simulink model "modelo_planta_sin_reference"  (R2023b)
settings: Solver=VariableStepAuto  StartTime=0.0  StopTime=50  RelTol=1e-3
undefined symbols (not defined in the file): ah_max, at_max, bcx, bcy, bhb, bhd, bhEb, bhm, bhwu, bt, btb, btd, btm, btw, DiscIntNeverNeededParam, g, h_vec, Hc, ih, it, J_hd_hEb, J_hm_hb, Jtd, Jtm_tb, Kcy, khwu, Ki_v, Kp_v, Kp_x, Ktw, Lh0, lh_0, M_base, magnitude, Mc_max, Ms, Mt, N_h, omega_h, P_nom, rhd, rtd, tau_hm, tau_tm, Thb_Max, ThEb_Max, Thm_0, Thm_Max, titahm_0, titatm_0, Ts2, Ttb_Max, Ttm_0, Ttm_Max, vh_max_unloaded, vlx_0, vly_0, vt_0, vt_max, Wc ... (+15)
libraries: simulink x12, simulink_extras x1
settings Model: Creator=Nahuel  LastModifiedBy=Nahuel

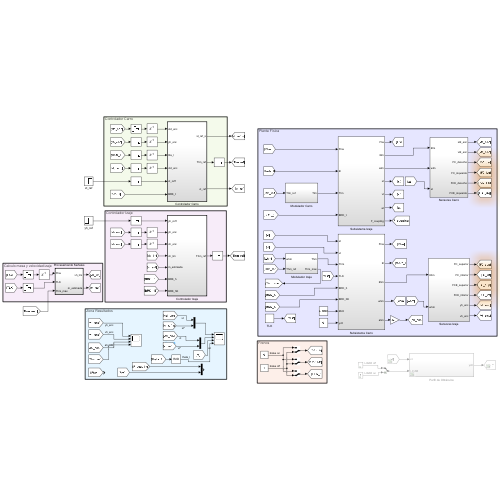
[thumbnail: Simulink's stored preview of the top-level diagram]
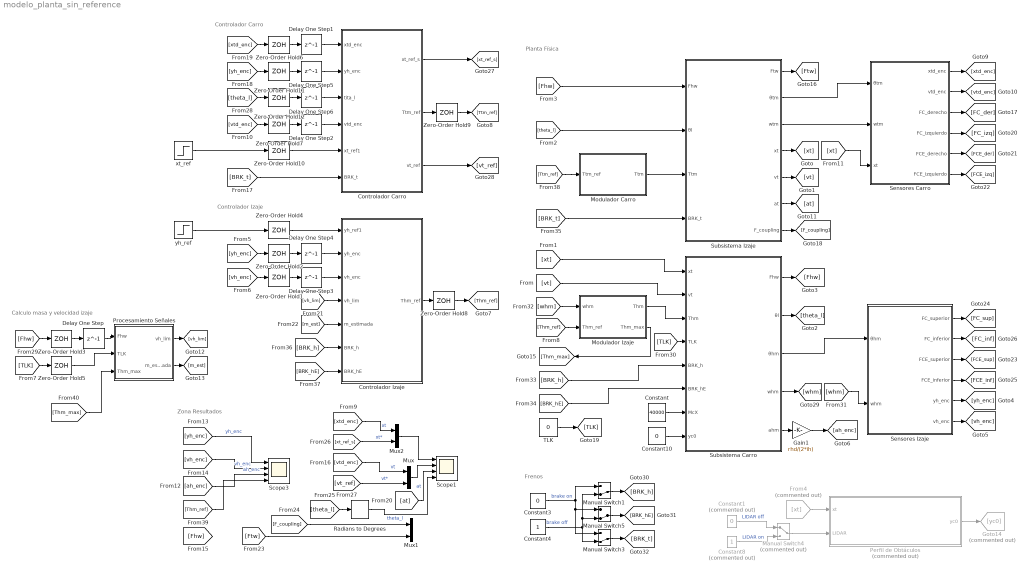
== system modelo_planta_sin_reference ==
  note: Frenos
  note: Controlador Izaje
  note: Calculo masa y velocidad izaje
  note: Controlador Carro
  note: Planta Física
  note: Zona Resultados
  Constant : Constant  Value=40000
  Constant1 : Constant  Commented=on  Value=0
  Constant10 : Constant  Value=0
  Constant3 : Constant  Value=0
  Constant4 : Constant
  Constant8 : Constant  Commented=on
  Controlador Carro : Subsystem  TreatAsAtomicUnit=on  SystemSampleTime=Ts2
  Controlador Izaje : Subsystem  TreatAsAtomicUnit=on  SystemSampleTime=Ts2
  Delay One Step : Delay  DelayLength=1
  Delay One Step1 : Delay  DelayLength=1  InitialCondition=xt_0
  Delay One Step2 : Delay  DelayLength=1  InitialCondition=vt_0
  Delay One Step3 : Delay  DelayLength=1  InitialCondition=whm_0
  Delay One Step4 : Delay  DelayLength=1  InitialCondition=yh_0
  Delay One Step5 : Delay  DelayLength=1  InitialCondition=yh_0
  Delay One Step6 : Delay  DelayLength=1  InitialCondition=0
  From4 : From  Commented=on  GotoTag=xt
  Gain1 : Gain  Gain=rhd/(2*ih)
  Goto14 : Goto  Commented=on  GotoTag=yc0
  Manual Switch1 : ManualSwitch  CurrentSetting=0
  Manual Switch3 : ManualSwitch  CurrentSetting=0
  Manual Switch4 : ManualSwitch  Commented=on
  Manual Switch5 : ManualSwitch  CurrentSetting=0
  Modulador Carro : Subsystem
  Modulador Izaje : Subsystem
  Mux : Mux  Inputs=2
  Mux1 : Mux  Inputs=2
  Mux2 : Mux  Inputs=2
  Perfil de Obtáculos : Subsystem  Commented=on
  Procesamiento Señales : Subsystem  TreatAsAtomicUnit=on  SystemSampleTime=Ts2
  Radians to Degrees : simulink_extras/Transformations/Radians to Degrees
  Scope1 : Scope  NumInputPorts=4
  Scope3 : Scope  NumInputPorts=4
  Sensores Carro : Subsystem
  Sensores Izaje : Subsystem
  Subsistema Carro : Subsystem
  Subsistema Izaje : Subsystem
  TLK : Constant  Value=0
  Zero-Order Hold{1..12} (12 alike) : ZeroOrderHold  SampleTime=Ts2
  xt_ref : Step  Time=0  Before=xt_0  After=0  SampleTime=0
  yh_ref : Step  Time=2  Before=yh_0  After=36.4  SampleTime=0
  wires:
  [Thm_ref] -> Modulador Izaje/2(Thm_ref)
  yh_ref/1 -> Zero-Order Hold4/1
  Constant1/1 -> Manual Switch4/1  "LIDAR off"
  [vt_ref] -> Mux/2  "vt*"
  Zero-Order Hold12/1 -> Delay One Step6/1
  [vh_enc] -> Scope3/2  "vh_enc"
  Sensores Izaje/2(FC_inferior) -> [FC_inf]
  [xt_ref_s] -> Mux2/2  "xt*"
  Controlador Carro/3(vt_ref) -> [vt_ref]
  xt_ref/1 -> Zero-Order Hold10/1
  Zero-Order Hold4/1 -> Controlador Izaje/1(yh_ref1)
  Delay One Step4/1 -> Controlador Izaje/2(yh_enc)
  Sensores Izaje/5(yh_enc) -> [yh_enc]
  [BRK_hE] -> Subsistema Carro/6(BRK_hE)
  Subsistema Carro/1(Fhw) -> [Fhw]
  [xtd_enc] -> Mux2/1  "xt"
  [vh_enc] -> Zero-Order Hold1/1
  Controlador Izaje/1(Thm_ref) -> Zero-Order Hold8/1
  Gain1/1 -> [ah_enc]
  Sensores Carro/1(xtd_enc) -> [xtd_enc]
  [yh_enc] -> Zero-Order Hold11/1
  Delay One Step6/1 -> Controlador Carro/3(tita_l)
  Zero-Order Hold11/1 -> Delay One Step5/1
  [xt] -> Sensores Carro/3(xt)
  [BRK_h] -> Subsistema Carro/5(BRK_h)
  [Ftw] -> Mux1/2
  Sensores Carro/4(FC_izquierdo) -> [FC_izq]
  [theta_l] -> Zero-Order Hold12/1
  Subsistema Carro/4(whm) -> [whm]
  Zero-Order Hold3/1 -> Delay One Step/1
  [m_est] -> Controlador Izaje/5(m_estimada)
  Controlador Carro/1(xt_ref_s) -> [xt_ref_s]
  Zero-Order Hold1/1 -> Delay One Step3/1
  Zero-Order Hold2/1 -> Delay One Step4/1
  Zero-Order Hold6/1 -> Delay One Step1/1
  Mux/1 -> Scope1/2
  Delay One Step/1 -> Procesamiento Señales/1(Fhw)
  Mux2/1 -> Scope1/1
  Subsistema Izaje/3(wtm) -> Sensores Carro/2(wtm)
  [Fhw] -> Zero-Order Hold3/1
  [at] -> Scope1/3  "at"
  Subsistema Izaje/6(at) -> [at]
  [vtd_enc] -> Mux/1  "vt"
  [theta_l] -> Subsistema Izaje/2(θl)
  [vt] -> Subsistema Carro/2(vt)
  [xt] -> Subsistema Carro/1(xt)
  Delay One Step1/1 -> Controlador Carro/1(xtd_enc)
  Procesamiento Señales/2(m_estimada) -> [m_est]
  [ah_enc] -> Scope3/3  "ah_enc"
  [vtd_enc] -> Zero-Order Hold7/1
  Subsistema Carro/5(ahm) -> Gain1/1
  Sensores Carro/2(vtd_enc) -> [vtd_enc]
  [TLK] -> Zero-Order Hold5/1
  Zero-Order Hold8/1 -> [Thm_ref]
  TLK/1 -> [TLK]
  Delay One Step3/1 -> Controlador Izaje/3(vh_enc)
  [vh_lim] -> Controlador Izaje/4(vh_lim)
  Subsistema Izaje/7(F_coupling) -> [F_coupling]
  Procesamiento Señales/1(vh_lim) -> [vh_lim]
  Zero-Order Hold5/1 -> Procesamiento Señales/2(TLK)
  Delay One Step2/1 -> Controlador Carro/4(vtd_enc)
  Zero-Order Hold10/1 -> Controlador Carro/5(xt_ref1)
  [theta_l] -> Radians to Degrees/1
  From4/1 -> Perfil de Obtáculos/1(xt)
  Subsistema Izaje/4(xt) -> [xt]
  [Fhw] -> Subsistema Izaje/1(Fhw)
  [F_coupling] -> Mux1/1
  Sensores Carro/6(FCE_izquierdo) -> [FCE_izq]
  [yh_enc] -> Zero-Order Hold2/1
  Perfil de Obtáculos/1(yc0) -> Goto14/1
  Sensores Izaje/6(vh_enc) -> [vh_enc]
  Constant8/1 -> Manual Switch4/2  "LIDAR on"
  [xtd_enc] -> Zero-Order Hold6/1
  Zero-Order Hold9/1 -> [Ttm_ref]
  Radians to Degrees/1 -> Scope1/4  "theta_l"
  Controlador Carro/2(Ttm_ref) -> Zero-Order Hold9/1
  [TLK] -> Subsistema Carro/4(TLK)
  Subsistema Carro/3(θhm) -> Sensores Izaje/1(θhm)
  Subsistema Izaje/2(θtm) -> Sensores Carro/1(θtm)
  Constant10/1 -> Subsistema Carro/8(yc0)
  Sensores Izaje/4(FCE_inferior) -> [FCE_inf]
  Sensores Izaje/3(FCE_superior) -> [FCE_sup]
  Sensores Izaje/1(FC_superior) -> [FC_sup]
  Manual Switch4/1 -> Perfil de Obtáculos/2(LIDAR)
  Sensores Carro/5(FCE_derecho) -> [FCE_der]
  Zero-Order Hold7/1 -> Delay One Step2/1
  Subsistema Carro/2(θl) -> [theta_l]
  Delay One Step5/1 -> Controlador Carro/2(yh_enc)
  Constant/1 -> Subsistema Carro/7(McX)
  Subsistema Izaje/5(vt) -> [vt]
  Sensores Carro/3(FC_derecho) -> [FC_der]
  Subsistema Izaje/1(Ftw) -> [Ftw]
  [whm] -> Sensores Izaje/2(whm)
  Constant3/1 -> Manual Switch3/1, Manual Switch5/1, Manual Switch1/1  "brake on"
  Constant4/1 -> Manual Switch1/2, Manual Switch5/2, Manual Switch3/2  "brake off"
  Manual Switch1/1 -> [BRK_h]
  Manual Switch5/1 -> [BRK_hE]
  Manual Switch3/1 -> [BRK_t]
  [BRK_t] -> Subsistema Izaje/4(BRK_t)
  [BRK_h] -> Controlador Izaje/6(BRK_h)
  [BRK_hE] -> Controlador Izaje/7(BRK_hE)
  [Ttm_ref] -> Modulador Carro/1(Ttm_ref)
  [BRK_t] -> Controlador Carro/6(BRK_t)
  [yh_enc] -> Scope3/1  "yh_enc"
  [whm] -> Modulador Izaje/1(whm)
  [Thm_ref] -> Scope3/4
  Modulador Carro/1(Ttm) -> Subsistema Izaje/3(Ttm)
  Modulador Izaje/2(Thm_max) -> [Thm_max]
  Modulador Izaje/1(Thm) -> Subsistema Carro/3(Thm)
  [Thm_max] -> Procesamiento Señales/3(Thm_max)

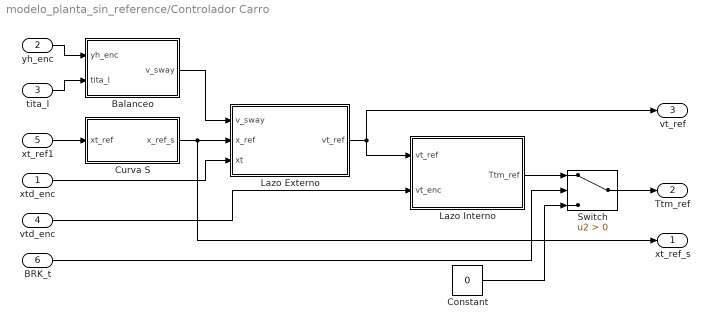
== system modelo_planta_sin_reference/Controlador Carro ==
  xtd_enc : Inport
  yh_enc : Inport  Port=2
  tita_l : Inport  Port=3
  vtd_enc : Inport  Port=4
  xt_ref1 : Inport  Port=5
  BRK_t : Inport  Port=6
  Balanceo : Subsystem
  Constant : Constant  Value=0
  Curva S : Subsystem
  Lazo Externo : Subsystem
  Lazo Interno : Subsystem
  Switch : Switch  Criteria=u2 > Threshold  SaturateOnIntegerOverflow=off  InputSameDT=off
  xt_ref_s : Outport
  Ttm_ref : Outport  Port=2
  vt_ref : Outport  Port=3
  wires:
  Lazo Externo/1(vt_ref) -> vt_ref/1, Lazo Interno/1(vt_ref)
  vtd_enc/1 -> Lazo Interno/2(vt_enc)
  xt_ref1/1 -> Curva S/1(xt_ref)
  Curva S/1(x_ref_s) -> xt_ref_s/1, Lazo Externo/2(x_ref)
  tita_l/1 -> Balanceo/2(tita_l)
  xtd_enc/1 -> Lazo Externo/3(xt)
  Balanceo/1(v_sway) -> Lazo Externo/1(v_sway)
  yh_enc/1 -> Balanceo/1(yh_enc)
  Switch/1 -> Ttm_ref/1
  BRK_t/1 -> Switch/2
  Lazo Interno/1(Ttm_ref) -> Switch/1
  Constant/1 -> Switch/3

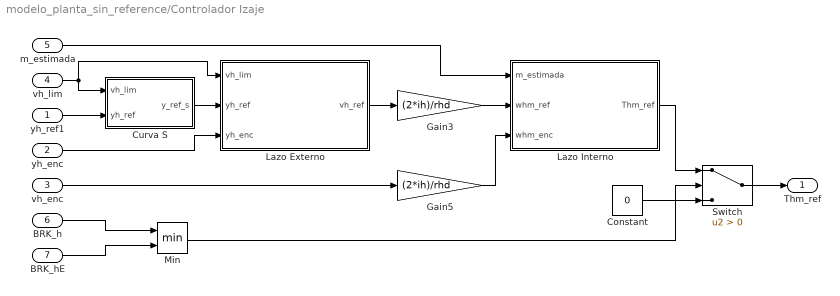
== system modelo_planta_sin_reference/Controlador Izaje ==
  yh_ref1 : Inport
  yh_enc : Inport  Port=2
  vh_enc : Inport  Port=3
  vh_lim : Inport  Port=4
  m_estimada : Inport  Port=5
  BRK_h : Inport  Port=6
  BRK_hE : Inport  Port=7
  Constant : Constant  Value=0
  Curva S : Subsystem
  Gain3 : Gain  Gain=(2*ih)/rhd
  Gain5 : Gain  Gain=(2*ih)/rhd
  Lazo Externo : Subsystem  TreatAsAtomicUnit=on  SystemSampleTime=Ts2
  Lazo Interno : Subsystem  TreatAsAtomicUnit=on  SystemSampleTime=Ts2
  Min : MinMax  Inputs=2
  Switch : Switch  Criteria=u2 > Threshold  SaturateOnIntegerOverflow=off  InputSameDT=off
  Thm_ref : Outport
  wires:
  Lazo Externo/1(vh_ref) -> Gain3/1
  m_estimada/1 -> Lazo Interno/1(m_estimada)
  vh_enc/1 -> Gain5/1
  yh_enc/1 -> Lazo Externo/3(yh_enc)
  Gain5/1 -> Lazo Interno/3(whm_enc)
  yh_ref1/1 -> Curva S/2(yh_ref)
  Gain3/1 -> Lazo Interno/2(whm_ref)
  Curva S/1(y_ref_s) -> Lazo Externo/2(yh_ref)
  BRK_h/1 -> Min/1
  BRK_hE/1 -> Min/2
  Min/1 -> Switch/2
  Switch/1 -> Thm_ref/1
  Lazo Interno/1(Thm_ref) -> Switch/1
  Constant/1 -> Switch/3
  vh_lim/1 -> Curva S/1(vh_lim), Lazo Externo/1(vh_lim)

== system modelo_planta_sin_reference/Modulador Carro ==
  Ttm_ref : Inport
  Constant : Constant  Value=Ttm_Max
  Gain1 : Gain  Gain=-1
  Gain2 : Gain  Gain=1/tau_tm
  Integrator : Integrator  InitialCondition=Ttm_0
  Saturation Dynamic : simulink/Discontinuities/Saturation Dynamic  OutMin=[]  OutMax=[]  OutDataTypeStr=Inherit: Same as second input  OutDataType=fixdt(1, 16)  OutScaling=2^-10  DoSatur=off
  Sum : Sum  Inputs=|+-
  Ttm : Outport
  wires:
  Constant/1 -> Saturation Dynamic/1, Gain1/1
  Gain1/1 -> Saturation Dynamic/3
  Saturation Dynamic/1 -> Sum/1  "Ttm_lim"
  Sum/1 -> Gain2/1
  Gain2/1 -> Integrator/1
  Integrator/1 -> Ttm/1, Sum/2
  Ttm_ref/1 -> Saturation Dynamic/2

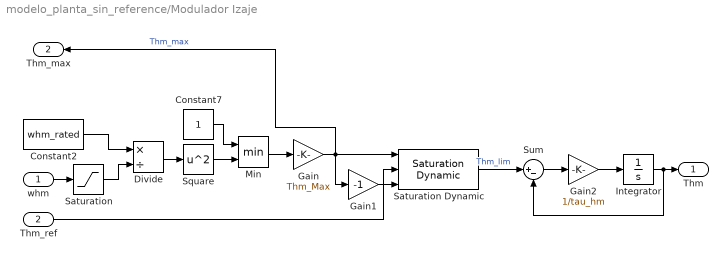
== system modelo_planta_sin_reference/Modulador Izaje ==
  whm : Inport
  Thm_ref : Inport  Port=2
  Constant2 : Constant  Value=whm_rated
  Constant7 : Constant
  Divide : Product  Inputs=*/
  Gain : Gain  Gain=Thm_Max
  Gain1 : Gain  Gain=-1
  Gain2 : Gain  Gain=1/tau_hm
  Integrator : Integrator  InitialCondition=Thm_0
  Min : MinMax  Inputs=2
  Saturation : Saturate  UpperLimit=inf  LowerLimit=whm_rated
  Saturation Dynamic : simulink/Discontinuities/Saturation Dynamic  OutMin=[]  OutMax=[]  OutDataTypeStr=Inherit: Same as second input  OutDataType=fixdt(1, 16)  OutScaling=2^-10  DoSatur=off
  Square : Math  Operator=square
  Sum : Sum  Inputs=|+-
  Thm : Outport
  Thm_max : Outport  Port=2
  wires:
  Constant2/1 -> Divide/1
  Min/1 -> Gain/1
  Constant7/1 -> Min/1
  Gain/1 -> Thm_max/1, Gain1/1, Saturation Dynamic/1  "Thm_max"
  Saturation/1 -> Divide/2
  Square/1 -> Min/2
  Divide/1 -> Square/1
  whm/1 -> Saturation/1
  Gain1/1 -> Saturation Dynamic/3
  Saturation Dynamic/1 -> Sum/1  "Thm_lim"
  Sum/1 -> Gain2/1
  Gain2/1 -> Integrator/1
  Integrator/1 -> Sum/2, Thm/1
  Thm_ref/1 -> Saturation Dynamic/2

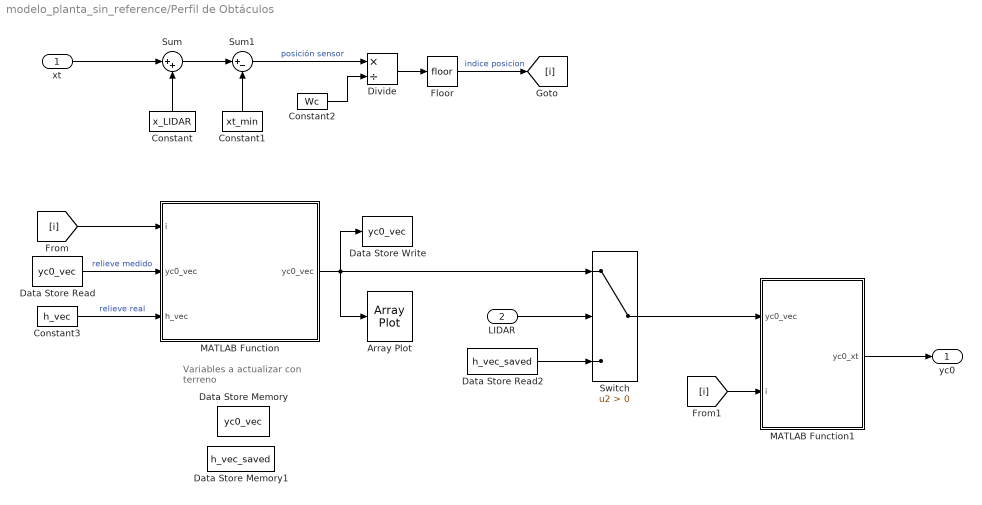
== system modelo_planta_sin_reference/Perfil de Obtáculos ==
  note: Variables a actualizar
      | con terreno
  xt : Inport
  LIDAR : Inport  Port=2
  Array Plot : ArrayPlot  WindowPosition=[1051.000000,310.000000,800.000000,459.000000,]  ScopeFrameLocation=window  YLimits=[-2.5 22.5]
  Constant : Constant  Value=x_LIDAR
  Constant1 : Constant  Value=xt_min
  Constant2 : Constant  Value=Wc
  Constant3 : Constant  Value=h_vec
  Data Store Memory : DataStoreMemory  DataStoreName=yc0_vec  WriteAfterWriteMsg=warning  InitialValue=yc0_vec  ShowAdditionalParam=off
  Data Store Memory1 : DataStoreMemory  DataStoreName=h_vec_saved  WriteAfterWriteMsg=warning  InitialValue=h_vec_saved  ShowAdditionalParam=off
  Data Store Read : DataStoreRead  DataStoreName=yc0_vec  IndexOptions=Index vector (dialog)  Indices=1  OutputSizes=1
  Data Store Read2 : DataStoreRead  DataStoreName=h_vec_saved  IndexOptions=Index vector (dialog)  Indices=1  OutputSizes=1
  Data Store Write : DataStoreWrite  DataStoreName=yc0_vec  IndexOptions=Index vector (dialog)  Indices=1  OutputSizes=1
  Divide : Product  Inputs=*/
  Floor : Rounding
  MATLAB Function : MATLAB Function  TreatAsAtomicUnit=on
  MATLAB Function1 : MATLAB Function  TreatAsAtomicUnit=on
  Sum : Sum  Inputs=|++
  Sum1 : Sum  Inputs=|+-
  Switch : Switch  Criteria=u2 > Threshold  SaturateOnIntegerOverflow=off  InputSameDT=off
  yc0 : Outport
  wires:
  xt/1 -> Sum/1
  Constant/1 -> Sum/2
  Sum/1 -> Sum1/1
  Constant1/1 -> Sum1/2
  Sum1/1 -> Divide/1  "posición sensor"
  Constant2/1 -> Divide/2
  Divide/1 -> Floor/1
  Data Store Read/1 -> MATLAB Function/2("yc0_vec ")  "relieve medido"
  MATLAB Function/1(yc0_vec) -> Array Plot/1, Data Store Write/1, Switch/1
  Constant3/1 -> MATLAB Function/3(h_vec)  "relieve real"
  LIDAR/1 -> Switch/2
  Data Store Read2/1 -> Switch/3
  Switch/1 -> MATLAB Function1/1(yc0_vec)
  MATLAB Function1/1(yc0_xt) -> yc0/1
  Floor/1 -> [i]  "indice posicion"
  [i] -> MATLAB Function/1(i)
  [i] -> MATLAB Function1/2(i)

== system modelo_planta_sin_reference/Procesamiento Señales ==
  Fhw : Inport
  TLK : Inport  Port=2
  Thm_max : Inport  Port=3
  Curva Potencia Original (no anda?) : MATLAB Function  TreatAsAtomicUnit=on
  Curva de Potencia : MATLAB Function  TreatAsAtomicUnit=on
  Estimación de Masa : Subsystem
  vh_lim : Outport
  m_estimada : Outport  Port=2
  wires:
  Estimación de Masa/1(m_estimada) -> Curva de Potencia/1(m_estimada), m_estimada/1
  TLK/1 -> Estimación de Masa/2(TLK)
  Fhw/1 -> Estimación de Masa/1(Fhw)
  Thm_max/1 -> Curva de Potencia/2(Thm_Max)
  Curva de Potencia/1(vh_lim) -> vh_lim/1

== system modelo_planta_sin_reference/Sensores Carro ==
  θtm : Inport
  wtm : Inport  Port=2
  xt : Inport  Port=3
  Encoder Carro : Subsystem
  Fines de carrera carro (rieles) : Subsystem
  xtd_enc : Outport
  vtd_enc : Outport  Port=2
  FC_derecho : Outport  Port=3
  FC_izquierdo : Outport  Port=4
  FCE_derecho : Outport  Port=5
  FCE_izquierdo : Outport  Port=6
  wires:
  Encoder Carro/1(xtd_enc) -> xtd_enc/1
  Fines de carrera carro (rieles)/1(FC_derecho) -> FC_derecho/1
  θtm/1 -> Encoder Carro/1(θtm)
  Fines de carrera carro (rieles)/2(FC_izquierdo) -> FC_izquierdo/1
  Encoder Carro/2(vtd_enc) -> vtd_enc/1
  Fines de carrera carro (rieles)/3(FCE_derecho) -> FCE_derecho/1
  Fines de carrera carro (rieles)/4(FCE_izquierdo) -> FCE_izquierdo/1
  xt/1 -> Fines de carrera carro (rieles)/1(xt)
  wtm/1 -> Encoder Carro/2(wtm)

== system modelo_planta_sin_reference/Sensores Izaje ==
  θhm : Inport
  whm : Inport  Port=2
  Encoder Izaje : Subsystem
  Fines de carrera izaje (tambor) : Subsystem
  FC_superior : Outport
  FC_inferior : Outport  Port=2
  FCE_superior : Outport  Port=3
  FCE_inferior : Outport  Port=4
  yh_enc : Outport  Port=5
  vh_enc : Outport  Port=6
  wires:
  Fines de carrera izaje (tambor)/1(FC_superior) -> FC_superior/1
  whm/1 -> Encoder Izaje/2(whm)
  Fines de carrera izaje (tambor)/4(FCE_inferior) -> FCE_inferior/1
  Fines de carrera izaje (tambor)/2(FC_inferior) -> FC_inferior/1
  Encoder Izaje/2(yh_enc) -> Fines de carrera izaje (tambor)/1(y_enc), yh_enc/1
  θhm/1 -> Encoder Izaje/1(θhm)
  Fines de carrera izaje (tambor)/3(FCE_superior) -> FCE_superior/1
  Encoder Izaje/1(vh_enc) -> vh_enc/1

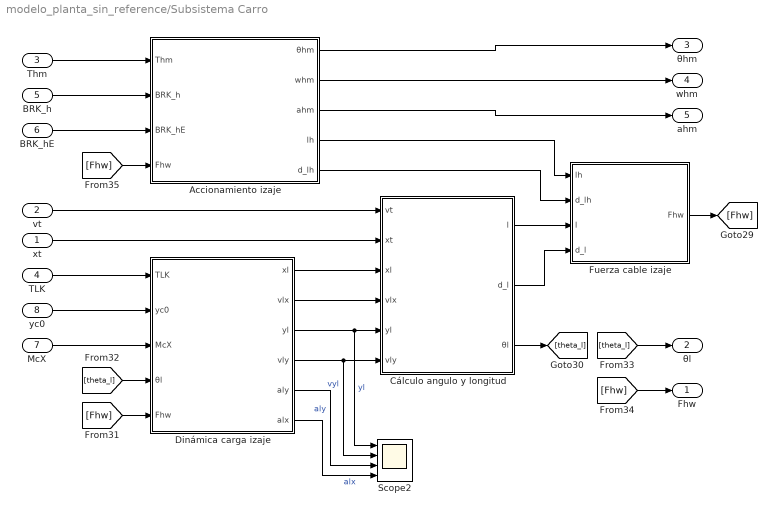
== system modelo_planta_sin_reference/Subsistema Carro ==
  xt : Inport
  vt : Inport  Port=2
  Thm : Inport  Port=3
  TLK : Inport  Port=4
  BRK_h : Inport  Port=5
  BRK_hE : Inport  Port=6
  McX : Inport  Port=7
  yc0 : Inport  Port=8
  Accionamiento izaje : Subsystem
  Cálculo angulo y longitud : Subsystem
  Dinámica carga izaje : Subsystem
  Fuerza cable izaje : Subsystem
  Scope2 : Scope  NumInputPorts=4
  Fhw : Outport
  θl : Outport  Port=2
  θhm : Outport  Port=3
  whm : Outport  Port=4
  ahm : Outport  Port=5
  wires:
  [Fhw] -> Fhw/1
  vt/1 -> Cálculo angulo y longitud/1(vt)
  Accionamiento izaje/4(lh) -> Fuerza cable izaje/1(lh)
  Dinámica carga izaje/5(aly) -> Scope2/3  "aly"
  yc0/1 -> Dinámica carga izaje/2(yc0)
  McX/1 -> Dinámica carga izaje/3(McX)
  Dinámica carga izaje/4(vly) -> Cálculo angulo y longitud/6(vly), Scope2/2  "vyl"
  [Fhw] -> Accionamiento izaje/4(Fhw)
  [theta_l] -> Dinámica carga izaje/4(θl)
  Cálculo angulo y longitud/3(θl) -> [theta_l]
  xt/1 -> Cálculo angulo y longitud/2(xt)
  BRK_h/1 -> Accionamiento izaje/2(BRK_h)
  Dinámica carga izaje/1(xl) -> Cálculo angulo y longitud/3(xl)
  Dinámica carga izaje/2(vlx) -> Cálculo angulo y longitud/4(vlx)
  Accionamiento izaje/3(ahm) -> ahm/1
  Dinámica carga izaje/6(alx) -> Scope2/4  "alx"
  Fuerza cable izaje/1(Fhw) -> [Fhw]
  Cálculo angulo y longitud/1(l) -> Fuerza cable izaje/3(l)
  Accionamiento izaje/1(θhm) -> θhm/1
  [theta_l] -> θl/1
  TLK/1 -> Dinámica carga izaje/1(TLK)
  [Fhw] -> Dinámica carga izaje/5(Fhw)
  Accionamiento izaje/2(whm) -> whm/1
  BRK_hE/1 -> Accionamiento izaje/3(BRK_hE)
  Thm/1 -> Accionamiento izaje/1(Thm)
  Dinámica carga izaje/3(yl) -> Cálculo angulo y longitud/5(yl), Scope2/1  "yl"
  Cálculo angulo y longitud/2(d_l) -> Fuerza cable izaje/4(d_l)
  Accionamiento izaje/5(d_lh) -> Fuerza cable izaje/2(d_lh)

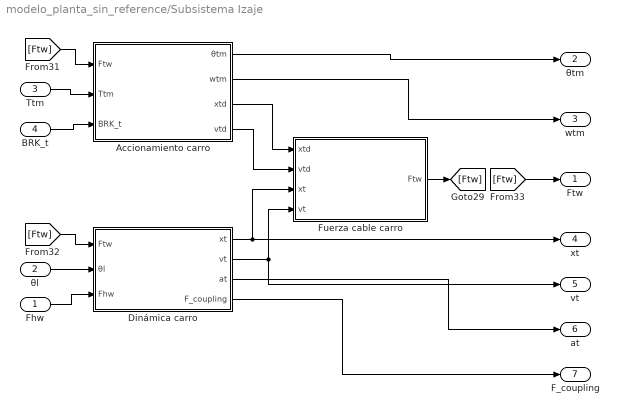
== system modelo_planta_sin_reference/Subsistema Izaje ==
  Fhw : Inport
  θl : Inport  Port=2
  Ttm : Inport  Port=3
  BRK_t : Inport  Port=4
  Accionamiento carro : Subsystem
  Dinámica carro : Subsystem
  Fuerza cable carro : Subsystem
  Ftw : Outport
  θtm : Outport  Port=2
  wtm : Outport  Port=3
  xt : Outport  Port=4
  vt : Outport  Port=5
  at : Outport  Port=6
  F_coupling : Outport  Port=7
  wires:
  [Ftw] -> Accionamiento carro/1(Ftw)
  Accionamiento carro/1(θtm) -> θtm/1
  Dinámica carro/1(xt) -> xt/1, Fuerza cable carro/3(xt)
  BRK_t/1 -> Accionamiento carro/3(BRK_t)
  [Ftw] -> Dinámica carro/1(Ftw)
  θl/1 -> Dinámica carro/2(θl)
  Ttm/1 -> Accionamiento carro/2(Ttm)
  Fuerza cable carro/1(Ftw) -> [Ftw]
  Dinámica carro/2(vt) -> vt/1, Fuerza cable carro/4(vt)
  Accionamiento carro/3(xtd) -> Fuerza cable carro/1(xtd)
  Dinámica carro/4(F_coupling) -> F_coupling/1
  Accionamiento carro/2(wtm) -> wtm/1
  Accionamiento carro/4(vtd) -> Fuerza cable carro/2(vtd)
  Fhw/1 -> Dinámica carro/3(Fhw)
  [Ftw] -> Ftw/1
  Dinámica carro/3(at) -> at/1

== system modelo_planta_sin_reference/Controlador Carro/Balanceo ==
  yh_enc : Inport
  tita_l : Inport  Port=2
  Constant9 : Constant  Value=Yt0
  Gain : Gain  Gain=g
  Gain1 : Gain  Gain=0.5
  Product : Product
  Saturation : Saturate  UpperLimit=vt_max/2  LowerLimit=-vt_max/2
  Sqrt : Sqrt
  Sum : Sum  Inputs=|+-
  v_sway : Outport
  wires:
  yh_enc/1 -> Sum/2
  Constant9/1 -> Sum/1
  Sum/1 -> Gain/1  "l"
  Gain/1 -> Sqrt/1
  Sqrt/1 -> Gain1/1
  Gain1/1 -> Product/2
  tita_l/1 -> Product/1
  Product/1 -> Saturation/1
  Saturation/1 -> v_sway/1

== system modelo_planta_sin_reference/Controlador Carro/Curva S ==
  xt_ref : Inport
  Delay : Delay  DelayLength=1  InitialCondition=xt_0
  Discrete-Time Integrator1 : DiscreteIntegrator  IntegratorMethod=Integration: Trapezoidal  InitialCondition=xt_0  SampleTime=-1  ICPrevOutput=DiscIntNeverNeededParam  ICPrevScaledInput=DiscIntNeverNeededParam
  MATLAB Function : MATLAB Function  TreatAsAtomicUnit=on
  Rate Limiter : RateLimiter  RisingSlewLimit=at_max  FallingSlewLimit=-at_max  SampleTimeMode=inherited
  Saturation : Saturate  UpperLimit=vt_max  LowerLimit=-vt_max
  Sum : Sum  Inputs=|+-
  x_ref_s : Outport
  wires:
  MATLAB Function/1(vt_cmd) -> Saturation/1  "vt_cmd"
  Discrete-Time Integrator1/1 -> x_ref_s/1, Delay/1
  Rate Limiter/1 -> Discrete-Time Integrator1/1
  Sum/1 -> MATLAB Function/1(error_pos)
  Saturation/1 -> Rate Limiter/1  "vt_ref"
  xt_ref/1 -> Sum/1
  Delay/1 -> Sum/2

== system modelo_planta_sin_reference/Controlador Carro/Lazo Externo ==
  v_sway : Inport
  x_ref : Inport  Port=2
  xt : Inport  Port=3
  Gain : Gain  Gain=Kp_x
  Rate Limiter : RateLimiter  RisingSlewLimit=at_max  FallingSlewLimit=-at_max  SampleTimeMode=inherited
  Saturation : Saturate  UpperLimit=vt_max  LowerLimit=-vt_max
  Sum : Sum  Inputs=|++
  Sum3 : Sum  Inputs=|+-
  vt_ref : Outport
  wires:
  xt/1 -> Sum3/2
  x_ref/1 -> Sum3/1
  Sum3/1 -> Gain/1  "e_x"
  Saturation/1 -> Rate Limiter/1
  v_sway/1 -> Sum/2
  Sum/1 -> Saturation/1
  Gain/1 -> Sum/1
  Rate Limiter/1 -> vt_ref/1

== system modelo_planta_sin_reference/Controlador Carro/Lazo Interno ==
  vt_ref : Inport
  vt_enc : Inport  Port=2
  Delay One Step : Delay  DelayLength=1
  Delay One Step1 : Delay  DelayLength=1
  Gain : Gain  Gain=Ts2/2
  Gain5 : Gain  Gain=Ki_v
  Gain6 : Gain  Gain=Kp_v
  Sum4 : Sum  Inputs=|++
  Sum5 : Sum  Inputs=|++
  Sum6 : Sum  Inputs=|+-
  Sum7 : Sum  Inputs=++|
  Ttm_ref : Outport
  wires:
  Sum6/1 -> Gain6/1, Sum4/1, Delay One Step/1  "e_v"
  Delay One Step/1 -> Sum4/2
  Sum5/1 -> Gain5/1, Delay One Step1/1
  Sum7/1 -> Ttm_ref/1
  Gain/1 -> Sum5/1
  Gain5/1 -> Sum7/2
  Delay One Step1/1 -> Sum5/2
  vt_ref/1 -> Sum6/1
  Gain6/1 -> Sum7/1
  Sum4/1 -> Gain/1
  vt_enc/1 -> Sum6/2

== system modelo_planta_sin_reference/Controlador Izaje/Curva S ==
  vh_lim : Inport
  yh_ref : Inport  Port=2
  Delay : Delay  DelayLength=1  InitialCondition=yh_0
  Discrete-Time Integrator : DiscreteIntegrator  IntegratorMethod=Integration: Trapezoidal  InitialCondition=yh_0  SampleTime=-1  ICPrevOutput=DiscIntNeverNeededParam  ICPrevScaledInput=DiscIntNeverNeededParam
  Gain1 : Gain  Gain=-1
  MATLAB Function : MATLAB Function  TreatAsAtomicUnit=on
  Rate Limiter : RateLimiter  RisingSlewLimit=ah_max  FallingSlewLimit=-ah_max  SampleTimeMode=inherited
  Saturation Dynamic : simulink/Discontinuities/Saturation Dynamic  OutMin=[]  OutMax=[]  OutDataTypeStr=Inherit: Same as second input  OutDataType=fixdt(1, 16)  OutScaling=2^-10  DoSatur=off
  Sum : Sum  Inputs=|+-
  y_ref_s : Outport
  wires:
  MATLAB Function/1(vh_cmd) -> Saturation Dynamic/2  "vh_cmd"
  Discrete-Time Integrator/1 -> Delay/1, y_ref_s/1
  Rate Limiter/1 -> Discrete-Time Integrator/1
  Sum/1 -> MATLAB Function/1(error_pos)
  vh_lim/1 -> Gain1/1, Saturation Dynamic/1
  Gain1/1 -> Saturation Dynamic/3
  Saturation Dynamic/1 -> Rate Limiter/1  "vh_ref"
  yh_ref/1 -> Sum/1
  Delay/1 -> Sum/2

== system modelo_planta_sin_reference/Controlador Izaje/Lazo Externo ==
  vh_lim : Inport
  yh_ref : Inport  Port=2
  yh_enc : Inport  Port=3
  Gain1 : Gain  Gain=-1
  Kpos : Gain  Gain=omega_h/N_h
  Rate Limiter : RateLimiter  RisingSlewLimit=ah_max  FallingSlewLimit=-ah_max  SampleTimeMode=inherited
  Saturation Dynamic : simulink/Discontinuities/Saturation Dynamic  OutMin=[]  OutMax=[]  OutDataTypeStr=Inherit: Same as second input  OutDataType=fixdt(1, 16)  OutScaling=2^-10  DoSatur=off
  Sum : Sum  Inputs=|+-
  vh_ref : Outport
  wires:
  yh_ref/1 -> Sum/1
  vh_lim/1 -> Saturation Dynamic/1, Gain1/1
  Gain1/1 -> Saturation Dynamic/3
  yh_enc/1 -> Sum/2
  Kpos/1 -> Saturation Dynamic/2  "vh_cmd"
  Sum/1 -> Kpos/1
  Saturation Dynamic/1 -> Rate Limiter/1  "vh_ref"
  Rate Limiter/1 -> vh_ref/1

== system modelo_planta_sin_reference/Controlador Izaje/Lazo Interno ==
  m_estimada : Inport
  whm_ref : Inport  Port=2
  whm_enc : Inport  Port=3
  Delay : Delay  DelayLength=1
  Delay1 : Delay  DelayLength=1
  Gain : Gain  Gain=Ts2/2
  Gain2 : Gain  Gain=g*rhd/(2*ih)
  Ki : Gain  Gain=(omega_h^2)*(J_hm_hb + (J_hd_hEb/(ih^2)))
  Kp : Gain  Gain=2*zitta_h*omega_h*(J_hm_hb + (J_hd_hEb/(ih^2)))
  Sum1 : Sum  Inputs=+-
  Sum{2..5} (4 alike) : Sum  Inputs=|++
  Thm_ref : Outport
  wires:
  Gain/1 -> Sum3/1
  Delay1/1 -> Sum3/2
  Kp/1 -> Sum4/1
  Sum1/1 -> Delay/1, Sum2/1, Kp/1  "e_wh"
  whm_enc/1 -> Sum1/2
  Sum3/1 -> Delay1/1, Ki/1
  Gain2/1 -> Sum5/2  "Tg_ff"
  Delay/1 -> Sum2/2
  Ki/1 -> Sum4/2
  Sum5/1 -> Thm_ref/1  "Thm_ref"
  Sum2/1 -> Gain/1
  Sum4/1 -> Sum5/1  "T_PID"
  whm_ref/1 -> Sum1/1
  m_estimada/1 -> Gain2/1

== system modelo_planta_sin_reference/Procesamiento Señales/Estimación de Masa ==
  Fhw : Inport
  TLK : Inport  Port=2
  Constant : Constant  Value=Ms
  Gain : Gain  Gain=2/g
  Switch : Switch  Criteria=u2 > Threshold  SaturateOnIntegerOverflow=off  InputSameDT=off
  m_estimada : Outport
  wires:
  Switch/1 -> m_estimada/1  "m_est"
  Gain/1 -> Switch/1
  Fhw/1 -> Gain/1
  Constant/1 -> Switch/3
  TLK/1 -> Switch/2

== system modelo_planta_sin_reference/Sensores Carro/Encoder Carro ==
  θtm : Inport
  wtm : Inport  Port=2
  Gain : Gain  Gain=rtd/it
  Gain1 : Gain  Gain=rtd/it
  xtd_enc : Outport
  vtd_enc : Outport  Port=2
  wires:
  Gain1/1 -> vtd_enc/1
  Gain/1 -> xtd_enc/1
  wtm/1 -> Gain1/1
  θtm/1 -> Gain/1

== system modelo_planta_sin_reference/Sensores Carro/Fines de carrera carro (rieles) ==
  xt : Inport
  Compare To Constant : simulink/Logic and Bit Operations/Compare To Constant  relop=>=  const=xt_max  OutDataTypeStr=boolean
  Compare To Constant1 : simulink/Logic and Bit Operations/Compare To Constant  relop=>=  const=xt_max+0.5  OutDataTypeStr=boolean
  Compare To Constant2 : simulink/Logic and Bit Operations/Compare To Constant  relop=<=  const=xt_min  OutDataTypeStr=boolean
  Compare To Constant3 : simulink/Logic and Bit Operations/Compare To Constant  relop=<=  const=xt_min-0.5  OutDataTypeStr=boolean
  FC_derecho : Outport
  FC_izquierdo : Outport  Port=2
  FCE_derecho : Outport  Port=3
  FCE_izquierdo : Outport  Port=4
  wires:
  Compare To Constant2/1 -> FC_izquierdo/1
  xt/1 -> Compare To Constant/1, Compare To Constant1/1, Compare To Constant2/1, Compare To Constant3/1
  Compare To Constant3/1 -> FCE_izquierdo/1
  Compare To Constant1/1 -> FCE_derecho/1
  Compare To Constant/1 -> FC_derecho/1

== system modelo_planta_sin_reference/Sensores Izaje/Encoder Izaje ==
  θhm : Inport
  whm : Inport  Port=2
  Gain1 : Gain  Gain=rhd/(2*ih)
  Gain3 : Gain  Gain=rhd/(2*ih)
  vh_enc : Outport
  yh_enc : Outport  Port=2
  wires:
  Gain1/1 -> vh_enc/1
  θhm/1 -> Gain3/1
  whm/1 -> Gain1/1
  Gain3/1 -> yh_enc/1

== system modelo_planta_sin_reference/Sensores Izaje/Fines de carrera izaje (tambor) ==
  y_enc : Inport
  Compare To Constant4 : simulink/Logic and Bit Operations/Compare To Constant  relop=>=  const=yh_max  OutDataTypeStr=boolean
  Compare To Constant5 : simulink/Logic and Bit Operations/Compare To Constant  relop=>=  const=yh_max+0.5  OutDataTypeStr=boolean
  Compare To Constant6 : simulink/Logic and Bit Operations/Compare To Constant  relop=<=  const=yh_min  OutDataTypeStr=boolean
  Compare To Constant7 : simulink/Logic and Bit Operations/Compare To Constant  relop=<=  const=yh_min-0.5  OutDataTypeStr=boolean
  FC_superior : Outport
  FC_inferior : Outport  Port=2
  FCE_superior : Outport  Port=3
  FCE_inferior : Outport  Port=4
  wires:
  Compare To Constant7/1 -> FCE_inferior/1
  y_enc/1 -> Compare To Constant7/1, Compare To Constant6/1, Compare To Constant4/1, Compare To Constant5/1
  Compare To Constant6/1 -> FC_inferior/1
  Compare To Constant5/1 -> FCE_superior/1
  Compare To Constant4/1 -> FC_superior/1

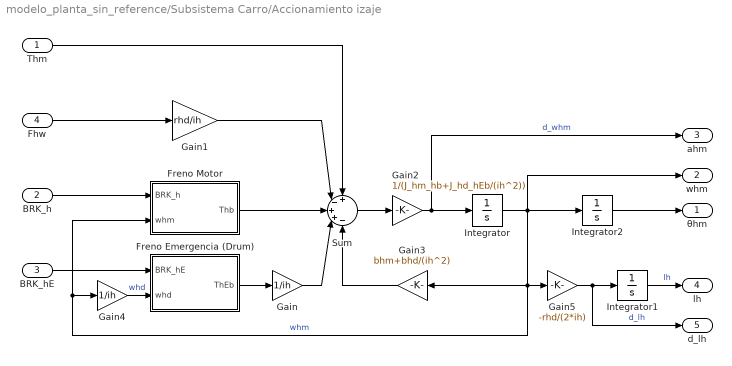
== system modelo_planta_sin_reference/Subsistema Carro/Accionamiento izaje ==
  Thm : Inport
  BRK_h : Inport  Port=2
  BRK_hE : Inport  Port=3
  Fhw : Inport  Port=4
  Freno Emergencia (Drum) : Subsystem
  Freno Motor : Subsystem
  Gain : Gain  Gain=1/ih
  Gain1 : Gain  Gain=rhd/ih
  Gain2 : Gain  Gain=1/(J_hm_hb+J_hd_hEb/(ih^2))
  Gain3 : Gain  Gain=bhm+bhd/(ih^2)
  Gain4 : Gain  Gain=1/ih
  Gain5 : Gain  Gain=-rhd/(2*ih)
  Integrator : Integrator  InitialCondition=whm_0
  Integrator1 : Integrator  InitialCondition=lh_0
  Integrator2 : Integrator  InitialCondition=titahm_0
  Sum : Sum  Inputs=+-++-
  θhm : Outport
  whm : Outport  Port=2
  ahm : Outport  Port=3
  lh : Outport  Port=4
  d_lh : Outport  Port=5
  wires:
  Gain5/1 -> d_lh/1, Integrator1/1  "d_lh"
  Integrator/1 -> Gain3/1, Freno Motor/2(whm), Gain4/1, Gain5/1, whm/1, Integrator2/1  "whm"
  Freno Emergencia (Drum)/1(ThEb) -> Gain/1
  Gain3/1 -> Sum/5
  BRK_h/1 -> Freno Motor/1(BRK_h)
  Gain/1 -> Sum/4
  Gain2/1 -> ahm/1, Integrator/1  "d_whm"
  Sum/1 -> Gain2/1
  Gain4/1 -> Freno Emergencia (Drum)/2(whd)  "whd"
  BRK_hE/1 -> Freno Emergencia (Drum)/1(BRK_hE)
  Fhw/1 -> Gain1/1
  Freno Motor/1(Thb) -> Sum/3
  Gain1/1 -> Sum/2
  Integrator1/1 -> lh/1  "lh"
  Integrator2/1 -> θhm/1
  Thm/1 -> Sum/1

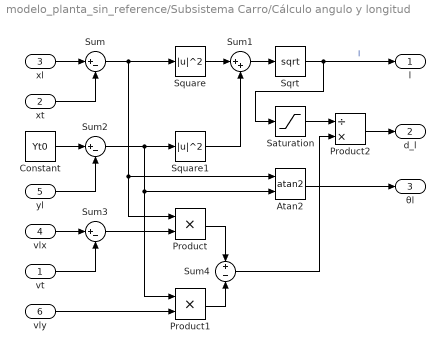
== system modelo_planta_sin_reference/Subsistema Carro/Cálculo angulo y longitud ==
  vt : Inport
  xt : Inport  Port=2
  xl : Inport  Port=3
  vlx : Inport  Port=4
  yl : Inport  Port=5
  vly : Inport  Port=6
  Atan2 : Trigonometry  Operator=atan2
  Constant : Constant  Value=Yt0
  Product : Product
  Product1 : Product
  Product2 : Product  Inputs=/*
  Saturation : Saturate  UpperLimit=inf  LowerLimit=0.1
  Sqrt : Sqrt
  Square : Math  Operator=magnitude^2
  Square1 : Math  Operator=magnitude^2
  Sum : Sum  Inputs=|+-
  Sum1 : Sum  Inputs=|++
  Sum2 : Sum  Inputs=|+-
  Sum3 : Sum  Inputs=|+-
  Sum4 : Sum  Inputs=+-
  l : Outport
  d_l : Outport  Port=2
  θl : Outport  Port=3
  wires:
  Product2/1 -> d_l/1
  Sqrt/1 -> l/1, Saturation/1  "l"
  Sum1/1 -> Sqrt/1
  Sum2/1 -> Product1/1, Atan2/2, Square1/1
  Sum/1 -> Product/1, Atan2/1, Square/1
  yl/1 -> Sum2/2
  Atan2/1 -> θl/1
  vly/1 -> Product1/2
  xl/1 -> Sum/1
  Constant/1 -> Sum2/1
  Sum3/1 -> Product/2
  Square1/1 -> Sum1/2
  vt/1 -> Sum3/2
  Sum4/1 -> Product2/2
  vlx/1 -> Sum3/1
  xt/1 -> Sum/2
  Square/1 -> Sum1/1
  Product1/1 -> Sum4/2
  Product/1 -> Sum4/1
  Saturation/1 -> Product2/1

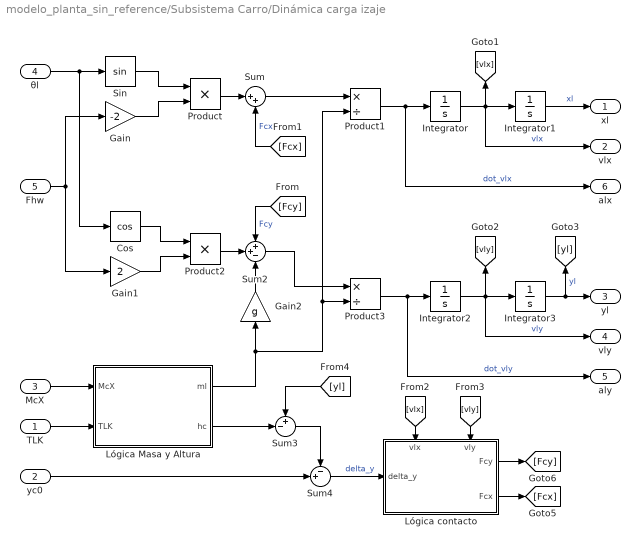
== system modelo_planta_sin_reference/Subsistema Carro/Dinámica carga izaje ==
  TLK : Inport
  yc0 : Inport  Port=2
  McX : Inport  Port=3
  θl : Inport  Port=4
  Fhw : Inport  Port=5
  Cos : Trigonometry  Operator=cos
  Gain : Gain  Gain=-2
  Gain1 : Gain  Gain=2
  Gain2 : Gain  Gain=g
  Integrator : Integrator  InitialCondition=vlx_0
  Integrator1 : Integrator  InitialCondition=xl_0
  Integrator2 : Integrator  InitialCondition=vly_0
  Integrator3 : Integrator  InitialCondition=yl_0
  Lógica Masa y Altura : Subsystem
  Lógica contacto : Subsystem
      settings: PortSchema="{\"entries\":[{\"content\":{\"sides\":[{\"content\":{\"connectorIds\":[\"In1\"]},\"type\":\"ConnectorPlacement.EquallySpacedRectSide\",\"uuid\":\"20a8b2c4-d5cf-44ce-93ec-929b996a0905\"},{\"content\":{\"connectorIds\":[\"Out1\",\"Out2\"],\"side\":\"RIGHT\"},\"type\":\"ConnectorPlacement.EquallySpacedRectSide\",\"uuid\":\"396e1f2e-cf71-48dc-8d57-a3e2695dfff1\"},{\"content\":{\"connectorIds\":[\"In2\",\"In3\"],\"side\":\"TOP\"},\"type\":\"ConnectorPlacement.EquallySpacedRectSide\",\"uuid\":\"e66c0478-9682-41e1-9b77-d2d789a9c323\"}]},\"type\":\"ConnectorPlacement.EquallySpacedConnector\",\"uuid\":\"193dabd2-f524-433a-b6ef-c1cab585578e\"}],\"packageUris\":[\"http://schema.mathworks.com/mf0/Connector/R2020b\"],\"version\":\"1.0\"}"
  Product : Product
  Product1 : Product  Inputs=*/
  Product2 : Product
  Product3 : Product  Inputs=*/
  Sin : Trigonometry
  Sum : Sum  Inputs=|++
  Sum2 : Sum  Inputs=++-
  Sum3 : Sum  Inputs=+-|
  Sum4 : Sum  Inputs=-+|
  xl : Outport
  vlx : Outport  Port=2
  yl : Outport  Port=3
  vly : Outport  Port=4
  aly : Outport  Port=5
  alx : Outport  Port=6
  wires:
  θl/1 -> Sin/1, Cos/1
  Integrator/1 -> vlx/1, Integrator1/1, [vlx]  "vlx"
  Sum3/1 -> Sum4/1
  Sin/1 -> Product/1
  Gain/1 -> Product/2
  [Fcy] -> Sum2/1  "Fcy"
  Integrator2/1 -> vly/1, Integrator3/1, [vly]  "vly"
  Integrator3/1 -> yl/1, [yl]  "yl"
  Fhw/1 -> Gain1/1, Gain/1
  [Fcx] -> Sum/2  "Fcx"
  Product/1 -> Sum/1
  Product1/1 -> alx/1, Integrator/1  "dot_vlx"
  Gain2/1 -> Sum2/3
  Cos/1 -> Product2/1
  Gain1/1 -> Product2/2
  [yl] -> Sum3/1
  Product2/1 -> Sum2/2
  yc0/1 -> Sum4/2
  Sum2/1 -> Product3/1
  Product3/1 -> aly/1, Integrator2/1  "dot_vly"
  Sum/1 -> Product1/1
  Integrator1/1 -> xl/1  "xl"
  Sum4/1 -> Lógica contacto/1(delta_y)  "delta_y"
  Lógica contacto/1(Fcy) -> [Fcy]
  Lógica contacto/2(Fcx) -> [Fcx]
  Lógica Masa y Altura/1(ml) -> Product1/2, Product3/2, Gain2/1
  McX/1 -> Lógica Masa y Altura/1(McX)
  TLK/1 -> Lógica Masa y Altura/2(TLK)
  Lógica Masa y Altura/2(hc) -> Sum3/2
  [vlx] -> Lógica contacto/2(vlx)
  [vly] -> Lógica contacto/3(vly)

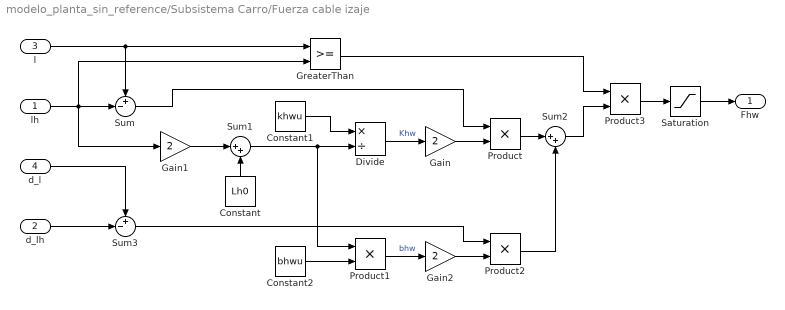
== system modelo_planta_sin_reference/Subsistema Carro/Fuerza cable izaje ==
  lh : Inport
  d_lh : Inport  Port=2
  l : Inport  Port=3
  d_l : Inport  Port=4
  Constant : Constant  Value=Lh0
  Constant1 : Constant  Value=khwu
  Constant2 : Constant  Value=bhwu
  Divide : Product  Inputs=*/  RndMeth=Zero  SaturateOnIntegerOverflow=on
  Gain : Gain  Gain=2
  Gain1 : Gain  Gain=2
  Gain2 : Gain  Gain=2
  GreaterThan : RelationalOperator  OutDataTypeStr=boolean  RndMeth=Simplest  InputSameDT=off
  Product{,1..3} (4 alike) : Product
  Saturation : Saturate  UpperLimit=inf  LowerLimit=0
  Sum : Sum  Inputs=+-|
  Sum1 : Sum  Inputs=|++
  Sum2 : Sum  Inputs=|++
  Sum3 : Sum  Inputs=+-|
  Fhw : Outport
  wires:
  Constant/1 -> Sum1/2
  Constant2/1 -> Product1/2
  Sum1/1 -> Divide/2, Product1/1
  lh/1 -> Sum/2, GreaterThan/2, Gain1/1
  Product/1 -> Sum2/1
  Gain1/1 -> Sum1/1
  l/1 -> Sum/1, GreaterThan/1
  Product2/1 -> Sum2/2
  Product3/1 -> Saturation/1
  GreaterThan/1 -> Product3/1
  d_lh/1 -> Sum3/2
  Constant1/1 -> Divide/1
  Product1/1 -> Gain2/1  "bhw"
  Sum/1 -> Product/1
  Gain2/1 -> Product2/2
  Divide/1 -> Gain/1  "Khw"
  Sum2/1 -> Product3/2
  Sum3/1 -> Product2/1
  d_l/1 -> Sum3/1
  Gain/1 -> Product/2
  Saturation/1 -> Fhw/1

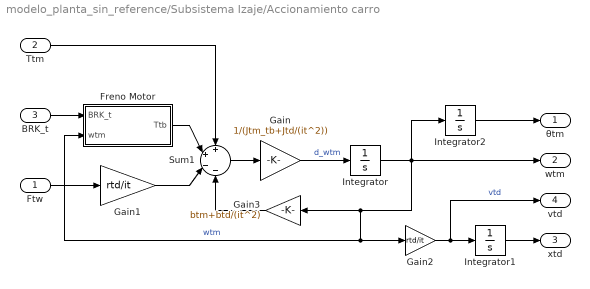
== system modelo_planta_sin_reference/Subsistema Izaje/Accionamiento carro ==
  Ftw : Inport
  Ttm : Inport  Port=2
  BRK_t : Inport  Port=3
  Freno Motor : Subsystem
  Gain : Gain  Gain=1/(Jtm_tb+Jtd/(it^2))
  Gain1 : Gain  Gain=rtd/it
  Gain2 : Gain  Gain=rtd/it
  Gain3 : Gain  Gain=btm+btd/(it^2)
  Integrator : Integrator  InitialCondition=wtm_0
  Integrator1 : Integrator  InitialCondition=xtd_0
  Integrator2 : Integrator  InitialCondition=titatm_0
  Sum1 : Sum  Inputs=++--
  θtm : Outport
  wtm : Outport  Port=2
  xtd : Outport  Port=3
  vtd : Outport  Port=4
  wires:
  Sum1/1 -> Gain/1
  Integrator/1 -> Gain2/1, Freno Motor/2(wtm), Gain3/1, Integrator2/1, wtm/1  "wtm"
  Gain2/1 -> Integrator1/1, vtd/1  "vtd"
  Ttm/1 -> Sum1/1
  Gain/1 -> Integrator/1  "d_wtm"
  BRK_t/1 -> Freno Motor/1(BRK_t)
  Integrator1/1 -> xtd/1
  Ftw/1 -> Gain1/1
  Gain1/1 -> Sum1/3
  Freno Motor/1(Ttb) -> Sum1/2
  Gain3/1 -> Sum1/4
  Integrator2/1 -> θtm/1

== system modelo_planta_sin_reference/Subsistema Izaje/Dinámica carro ==
  Ftw : Inport
  θl : Inport  Port=2
  Fhw : Inport  Port=3
  Gain : Gain  Gain=2
  Gain1 : Gain  Gain=1/Mt
  Gain2 : Gain  Gain=bt
  Integrator : Integrator  InitialCondition=vt_0
  Integrator1 : Integrator  InitialCondition=xt_0
  Product : Product
  Sin : Trigonometry
  Sum : Sum  Inputs=++-
  xt : Outport
  vt : Outport  Port=2
  at : Outport  Port=3
  F_coupling : Outport  Port=4
  wires:
  Gain1/1 -> at/1, Integrator/1  "dot_vt"
  Integrator/1 -> Gain2/1, vt/1, Integrator1/1  "vt"
  Gain2/1 -> Sum/3
  Sum/1 -> Gain1/1
  Integrator1/1 -> xt/1  "xt"
  Fhw/1 -> Gain/1
  Gain/1 -> Product/2
  θl/1 -> Sin/1
  Sin/1 -> Product/1
  Product/1 -> F_coupling/1, Sum/2  "F_coupling"
  Ftw/1 -> Sum/1

== system modelo_planta_sin_reference/Subsistema Izaje/Fuerza cable carro ==
  xtd : Inport
  vtd : Inport  Port=2
  xt : Inport  Port=3
  vt : Inport  Port=4
  Gain : Gain  Gain=Ktw
  Gain1 : Gain  Gain=btw
  Sum : Sum  Inputs=+-
  Sum1 : Sum
  Sum2 : Sum  Inputs=+-
  Ftw : Outport
  wires:
  xtd/1 -> Sum/1
  Gain1/1 -> Sum1/2
  Sum/1 -> Gain/1
  xt/1 -> Sum/2
  Sum2/1 -> Gain1/1
  Gain/1 -> Sum1/1
  vt/1 -> Sum2/2
  Sum1/1 -> Ftw/1  "Ftw"
  vtd/1 -> Sum2/1

== system modelo_planta_sin_reference/Subsistema Carro/Accionamiento izaje/Freno Emergencia (Drum) ==
  BRK_hE : Inport
  whd : Inport  Port=2
  Constant : Constant  Value=0
  Gain3 : Gain  Gain=-ThEb_Max
  Gain4 : Gain  Gain=bhEb
  Switch : Switch  Criteria=u2 > Threshold  SaturateOnIntegerOverflow=off  InputSameDT=off
  Tanh : Trigonometry  Operator=tanh
  ThEb : Outport
  wires:
  BRK_hE/1 -> Switch/2
  Gain3/1 -> Switch/3
  Constant/1 -> Switch/1
  whd/1 -> Gain4/1
  Gain4/1 -> Tanh/1
  Tanh/1 -> Gain3/1
  Switch/1 -> ThEb/1

== system modelo_planta_sin_reference/Subsistema Carro/Accionamiento izaje/Freno Motor ==
  BRK_h : Inport
  whm : Inport  Port=2
  Constant : Constant  Value=0
  Gain3 : Gain  Gain=-Thb_Max
  Gain4 : Gain  Gain=bhb
  Switch : Switch  Criteria=u2 > Threshold  SaturateOnIntegerOverflow=off  InputSameDT=off
  Tanh : Trigonometry  Operator=tanh
  Thb : Outport
  wires:
  BRK_h/1 -> Switch/2
  Gain3/1 -> Switch/3
  Constant/1 -> Switch/1
  whm/1 -> Gain4/1
  Gain4/1 -> Tanh/1
  Tanh/1 -> Gain3/1
  Switch/1 -> Thb/1

== system modelo_planta_sin_reference/Subsistema Carro/Dinámica carga izaje/Lógica Masa y Altura ==
  McX : Inport
  TLK : Inport  Port=2
  Constant : Constant  Value=Ms
  Constant1 : Constant  Value=0
  Constant2 : Constant  Value=Hc
  Rate Limiter : RateLimiter  RisingSlewLimit=Mc_max/0.1  FallingSlewLimit=-Mc_max/0.1  SampleTimeMode=inherited  InitialCondition=Ms
  Sum1 : Sum  Inputs=|++
  Switch : Switch  Criteria=u2 > Threshold  SaturateOnIntegerOverflow=off  InputSameDT=off
  Switch1 : Switch  Criteria=u2 > Threshold  SaturateOnIntegerOverflow=off  InputSameDT=off
  ml : Outport
  hc : Outport  Port=2
  wires:
  Sum1/1 -> Switch/1
  Constant2/1 -> Switch1/1
  TLK/1 -> Switch1/2, Switch/2
  Constant/1 -> Switch/3, Sum1/2
  Constant1/1 -> Switch1/3
  McX/1 -> Sum1/1
  Switch/1 -> Rate Limiter/1
  Rate Limiter/1 -> ml/1
  Switch1/1 -> hc/1

== system modelo_planta_sin_reference/Subsistema Carro/Dinámica carga izaje/Lógica contacto ==
  delta_y : Inport
  vlx : Inport  Port=2
  vly : Inport  Port=3
  Constant3 : Constant  Value=0
  Constant4 : Constant  Value=0
  Gain3 : Gain  Gain=Kcy
  Gain4 : Gain  Gain=bcy
  Gain5 : Gain  Gain=-bcx
  Saturation : Saturate  UpperLimit=inf  LowerLimit=0
  Sum5 : Sum  Inputs=-+|
  Switch2 : Switch  SaturateOnIntegerOverflow=off  InputSameDT=off
  Switch3 : Switch  SaturateOnIntegerOverflow=off  InputSameDT=off
  Fcy : Outport
  Fcx : Outport  Port=2
  wires:
  Sum5/1 -> Switch2/1
  vlx/1 -> Gain5/1
  Gain4/1 -> Sum5/1
  vly/1 -> Gain4/1
  Constant4/1 -> Switch3/3
  Gain5/1 -> Switch3/1
  Gain3/1 -> Sum5/2
  delta_y/1 -> Switch3/2, Gain3/1, Switch2/2
  Constant3/1 -> Switch2/3
  Switch2/1 -> Saturation/1  "Fcy"
  Switch3/1 -> Fcx/1  "Fcx"
  Saturation/1 -> Fcy/1

== system modelo_planta_sin_reference/Subsistema Izaje/Accionamiento carro/Freno Motor ==
  BRK_t : Inport
  wtm : Inport  Port=2
  Constant : Constant  Value=0
  Gain3 : Gain  Gain=-Ttb_Max
  Gain4 : Gain  Gain=btb
  Switch : Switch  Criteria=u2 > Threshold  SaturateOnIntegerOverflow=off  InputSameDT=off
  Tanh : Trigonometry  Operator=tanh
  Ttb : Outport
  wires:
  BRK_t/1 -> Switch/2
  Constant/1 -> Switch/1
  wtm/1 -> Gain4/1
  Gain4/1 -> Tanh/1
  Tanh/1 -> Gain3/1
  Gain3/1 -> Switch/3
  Switch/1 -> Ttb/1

== matlab function modelo_planta_sin_reference/Perfil de Obtáculos/MATLAB Function1 ==
  data: yc0_vec input; yc0_xt output; i input
function yc0_xt = Calculo_yc0(yc0_vec,i)

yc0_xt = yc0_vec(i);

== matlab function modelo_planta_sin_reference/Perfil de Obtáculos/MATLAB Function ==
  data: i input; yc0_vec input; yc0_vec output; h_vec input
function yc0_vec  = actualizarPerfilObstaculos(i, yc0_vec, h_vec)
if(i<=33)
    yc0_vec(i) = h_vec(i);
end
end

== matlab function modelo_planta_sin_reference/Procesamiento Señales/Curva de Potencia ==
  data: m_estimada input; vh_lim output; g parameter; vh_max_unloaded parameter; rhd parameter; ih parameter; Thm_Max input
function vh_lim = fcn(m_estimada, g, vh_max_unloaded, rhd, ih, Thm_Max)
    % --- PARÁMETROS FIJOS ---
    % Velocidad lineal donde empieza el debilitamiento de campo (1.5 m/s)
    v_base = 1.5; 
    
    % --- 1. CALCULAR TORQUE REQUERIDO (CARGA) ---
    % Protegemos contra masa negativa o cero
    m_safe = max(m_estimada, 100); 
    
    % Fuerza en el cable
    F_cable = m_safe * g; 
    
    % Torque reflejado en el eje del motor (considerando reducción y eficiencia)
    T_load_motor = (F_cable * rhd) / (2*ih);

    % --- 2. CÁLCULO DEL LÍMITE DE VELOCIDAD ---
    % Ecuación: T_disp = T_max * (v_base / v_lim)^2
    % Despejamos v_lim cuando T_disp == T_load_motor
    
    if T_load_motor > Thm_Max
        % Si el torque necesario es mayor al máximo absoluto del motor:
        vh_lim = 0.0; % No se puede mover
    else
        % Despeje exacto: v_lim = v_base * sqrt( T_max / T_load )
        vh_calc = v_base * sqrt(Thm_Max / T_load_motor);
        
        % Saturamos con la velocidad mecánica máxima permitida
        vh_lim = min(vh_max_unloaded, vh_calc);
    end
end

== matlab function modelo_planta_sin_reference/Controlador Carro/Curva S/MATLAB Function ==
  data: error_pos input; vt_cmd output; at_max parameter
function vt_cmd = Frenado_OptimoT(error_pos, at_max)
    % Parámetro de suavizado (región lineal)
    d_tol = 0.1; % 10 cm de tolerancia donde se vuelve lineal
    
    if abs(error_pos) > d_tol
        % ZONA PARABÓLICA (Frenado Óptimo)
        % Lejos del objetivo, usamos la raíz cuadrada
        vh_brakes = sqrt(2 * at_max * abs(error_pos));
        vt_cmd = vh_brakes * sign(error_pos);
    else
        % ZONA LINEAL (Aterrizaje Suave)
        % Cerca del cero, usamos una ganancia fija para evitar pendiente infinita.
        vh_limit_tol = sqrt(2 * at_max * d_tol); % Velocidad en el borde de la zona
        gain_linear = vh_limit_tol / d_tol;      % Pendiente equivalente        
        vt_cmd = gain_linear * error_pos;
    end
end

== matlab function modelo_planta_sin_reference/Controlador Izaje/Curva S/MATLAB Function ==
  data: error_pos input; vh_cmd output; ah_max parameter
function vh_cmd = Frenado_Optimo(error_pos, ah_max)
    % Parámetro de suavizado (región lineal)
    d_tol = 0.1; % 10 cm de tolerancia donde se vuelve lineal
    
    if abs(error_pos) > d_tol
        % ZONA PARABÓLICA (Frenado Óptimo)
        % Lejos del objetivo, usamos la raíz cuadrada
        vh_brakes = sqrt(2 * ah_max * abs(error_pos));
        vh_cmd = vh_brakes * sign(error_pos);
    else
        % ZONA LINEAL (Aterrizaje Suave)
        % Cerca del cero, usamos una ganancia fija para evitar pendiente infinita.
        vh_limit_tol = sqrt(2 * ah_max * d_tol); % Velocidad en el borde de la zona
        gain_linear = vh_limit_tol / d_tol;      % Pendiente equivalente        
        vh_cmd = gain_linear * error_pos;
    end
end

== matlab function modelo_planta_sin_reference/Procesamiento Señales/Curva Potencia Original (no anda?) ==
  data: m_estimada input; vh_lim output; g parameter; vh_max_unloaded parameter; M_base parameter; P_nom parameter
function vh_lim = fcn(m_estimada, g, vh_max_unloaded, M_base, P_nom)
    % Implementación de la curva de potencia constante
    
    % Protección contra valores cero o negativos
    m_safe = max(m_estimada, 1000); 
    
    if m_safe < M_base
        % Zona de Velocidad Máxima Constante
        vh_lim = vh_max_unloaded;
    else
        % Zona de Potencia Constante (Hipérbola)
        vh_lim = P_nom / (m_safe * g);
    end
end
